simulink model "COMPoseTesting"  (Simulink 7.9)
settings: Solver=ode3  StartTime=0.0  StopTime=inf  FixedStep=Ts  RelTol=1e-3
libraries: WBCLibrary x1, simulink x1
settings Model: Creator=jorhabib  LastModifiedBy=daniele
settings CodeAppCC: CustomSymbolStrType=$N$R$M_T
settings GRTTargetCC: CodeReplacementLibrary=None  CPPClassGenCompliant=on

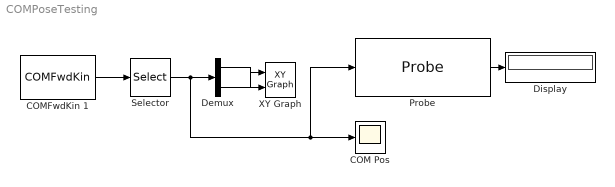
== system COMPoseTesting ==
  COM Pos : Scope
      settings: TimeRange=500  YMin=-0.07  YMax=0.07
  COMFwdKin 1 : WBCLibrary/wholeBodyModel/Forward Kinematics/COMFwdKin   robotName=robotName  localName=localName
  Demux : Demux  Outputs=2
  Display : Display
  Probe : Probe  ProbeWidth=off  ProbeComplexSignal=off
  Selector : Selector  InputPortWidth=7  IndexOptions=Index vector (dialog)  Indices=[1:2]  OutputSizes=1
  XY Graph : simulink/Sinks/XY Graph  xmin=-0.1  xmax=0.01  ymin=-0.05  ymax=0.05  st=-1
  wires:
  COMFwdKin 1/1 -> Selector/1
  Selector/1 -> Demux/1, COM Pos/1, Probe/1
  Demux/2 -> XY Graph/1
  Demux/1 -> XY Graph/2
  Probe/1 -> Display/1
